simulink model "power_monophaseline"  (Simulink 6.0)
settings: Solver=ode23tb  SolverMode=SingleTasking  StartTime=0.0  StopTime=0.1  RelTol=1e-5  AbsTol=1e-5
libraries: powerlib x17
settings Model: Creator=patrice  LastModifiedBy=batserve  ExtModeTrigMode=oneshot  ExtModeArmWhenConnect=off  ExtModeAutoUpdateStatusClock=off
settings DataIOCC: LimitDataPoints=off  SaveOutput=off  SaveTime=off  SignalLoggingName=sigsOut
settings OptimizationCC: BlockReduction=off  BooleanDataType=off
settings DebuggingCC: CheckExecutionContextPreStartOutputMsg=on  CheckExecutionContextRuntimeOutputMsg=on  SolverPrmCheckMsg=none  IntegerOverflowMsg=none
settings HardwareCC: TargetUnknown=on
settings RTWCC: TemplateMakefile=grt_unix.tmf

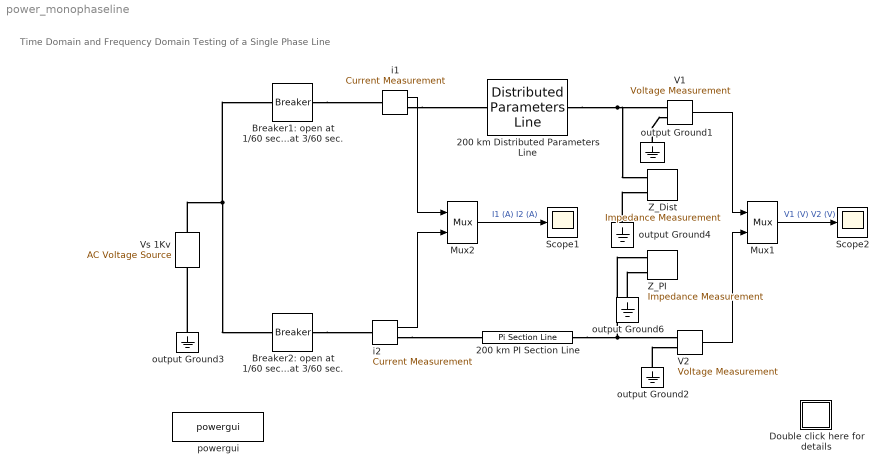
== system power_monophaseline ==
  note: Time Domain and Frequency Domain Testing of a Single Phase Line
  200 km Distributed Parameters Line : powerlib/Elements/Distributed Parameters Line  Phases=1  Frequency=60  Resistance=0.0955  Inductance=2.137e-3  Capacitance=12.37e-9  Length=200  x1=[0 -378.111478683995;0.000205658707571549 -305.271981817252;0.000411317415143098 -230.598373057679;0.000616976122714648 -154.539300699466;0.000822634830286197 -77.5517370737755;0.00102829353785775 -0.0982330023556983]  x2=[0 -417.766377531924;0.000205658707571549 -339.363445347372;0.000411317415143098 -258.921575532847;0.000616976122714648 -176.9240728097;0.000822634830286197 -93.8635883345532;0.00102829353785775 -10.2391597901105]  x3=[0 -1.7651045305041;0.000205658707571549 -1.62172775369337;0.000411317415143098 -1.4686074355911;0.000616976122714648 -1.30666354204152;0.000822634830286197 -1.13686905202344;0.00102829353785775 -0.960244111872024]  x4=[0 -0.971127277857831;0.000205658707571549 -0.788874156966986;0.000411317415143098 -0.601881382392148;0.000616976122714648 -0.411272429893128;0.000822634830286197 -0.218192501674784;0.00102829353785775 -0.0238016458702721]  x5=0.00102829353785775  Measurements=None
      settings: AttributesFormatString=\n
  200 km PI Section Line : powerlib/Elements/Pi Section Line  PhysicalDomain=powersysdomain  SubClassName=unknown  LeftPortType=p1  RightPortType=p1  LConnTagsString=__new0  RConnTagsString=__new0  Frequency=60  Resistance=0.0955  Inductance=2.137e-03  Capacitance=12.37e-09  Length=200  PiSections=2  Measurements=None
      settings: AttributesFormatString=\n
  Breaker1: open at 1/60 sec.  close at 3/60 sec. : powerlib/Elements/Breaker  BreakerResistance=0.1  InitialState=1  SnubberResistance=inf  SnubberCapacitance=0  SwitchingTimes="[ 1/60  3/60 ]"  External=off  Measurements=None
      settings: AttributesFormatString=\n
  Breaker2: open at 1/60 sec. close at 3/60 sec. : powerlib/Elements/Breaker  BreakerResistance=0.1  InitialState=1  SnubberResistance=inf  SnubberCapacitance=0  SwitchingTimes="[ 1/60  3/60 ]"  External=off  Measurements=None
      settings: AttributesFormatString=\n
  Double click here for details : Subsystem
      mask Display: disp('?')
  Mux1 : Mux  Inputs=2
  Mux2 : Mux  Inputs=2
  Scope1 : Scope
      settings: TickLabels=on  TimeRange=0.1  YMin=-4  YMax=4  DataFormat=Array
  Scope2 : Scope
      settings: TickLabels=on  TimeRange=0.1  YMin=-2500  YMax=2500  DataFormat=Array
  V1 : powerlib/Measurements/Voltage Measurement  Tag=PoWeRsYsTeMmEaSuReMeNt  PhasorSimulation=off  OutputType=Magnitude  PSBequivalent=0
  V2 : powerlib/Measurements/Voltage Measurement  Tag=PoWeRsYsTeMmEaSuReMeNt  PhasorSimulation=off  OutputType=Magnitude  PSBequivalent=0
  Vs 1Kv : powerlib/Electrical Sources/AC Voltage Source  Description=source block  Orientation=up  Amplitude=1e3  Phase=0  Frequency=60  SampleTime=0  Measurements=None
      settings: AttributesFormatString=\n
  Z_Dist : powerlib/Measurements/Impedance Measurement  PhysicalDomain=powersysdomain  SubClassName=unknown  LeftPortType=p1  RightPortType=p1  LConnTagsString=+|-  Factor=1
      settings: AttributesFormatString=\n
  Z_PI : powerlib/Measurements/Impedance Measurement  PhysicalDomain=powersysdomain  SubClassName=unknown  LeftPortType=p1  RightPortType=p1  LConnTagsString=+|-  Factor=1
      settings: AttributesFormatString=\n
  i1 : powerlib/Measurements/Current Measurement  Tag=PoWeRsYsTeMmEaSuReMeNt  PhasorSimulation=off  OutputType=Magnitude  PSBequivalent=0
  i2 : powerlib/Measurements/Current Measurement  Tag=PoWeRsYsTeMmEaSuReMeNt  PhasorSimulation=off  OutputType=Magnitude  PSBequivalent=0
  output Ground{1..4,6} (5 alike) : powerlib/Elements/Ground  Orientation=down  PhysicalDomain=powersysdomain  SubClassName=unknown  LeftPortType=p1  RightPortType=p1  LConnTagsString=a
  powergui : powerlib/powergui  Priority=2  Frange=0:2:2000  Ylog=on  Xlog=off  save=off  variable=ZData  ZoomFFT=on  StartTime=0.0  cycles=1  DisplayStyle=off  fundamental=60  FreqAxis=off  MaxFrequency=1000  frequencyindice=1  frequencyindicesteady=1  RmsSteady=1  display=on  Ts=0  methode=off  frequency=60  echomessages=on
  wires:
  Mux1/1 -> Scope2/1  "V1 (V) V2 (V)"
  Mux2/1 -> Scope1/1  "I1 (A) I2 (A)"
  i1/1 -> Mux2/1
  i2/1 -> Mux2/2
  V1/1 -> Mux1/1
  V2/1 -> Mux1/2
  connections:
  Breaker1: open at 1/60 sec.  close at 3/60 sec./RConn1 -- i1/LConn1
  i1/RConn1 -- 200 km Distributed Parameters Line/LConn1
  output Ground1/LConn1 -- V1/LConn2
  output Ground2/LConn1 -- V2/LConn2
  Breaker2: open at 1/60 sec. close at 3/60 sec./RConn1 -- i2/LConn1
  i2/RConn1 -- 200 km PI Section Line/LConn1
  output Ground3/LConn1 -- Vs 1Kv/LConn1
  Vs 1Kv/RConn1 -- Breaker1: open at 1/60 sec.  close at 3/60 sec./LConn1 -- Breaker2: open at 1/60 sec. close at 3/60 sec./LConn1
  200 km Distributed Parameters Line/RConn1 -- V1/LConn1 -- Z_Dist/LConn1
  output Ground4/LConn1 -- Z_Dist/LConn2
  output Ground6/LConn1 -- Z_PI/LConn2
  200 km PI Section Line/RConn1 -- V2/LConn1 -- Z_PI/LConn1

== system power_monophaseline/Double click here for details ==
  note: A  200 km line is connected on a 1 kV, 60 Hz  infinite source. The line is deenergized and then reenergized after 2 cycles.
      | The simulation is performed simultaneously with two different line models:
      |
      | - Distributed parameter line
      | - PI  section line consisting of two 100 km sections.
      |
      | Currents at the sending end and voltages at the receiving end are compared for the two line models.
      | Impedance Measurement blocks are connected at the open end of both  lines in order  to compare their frequency responses.
  note: Open the two scopes and start the simulation.
      | Observe the difference in current and voltage waveforms at breaker opening and reclosing.
      | Note the sharp edges of the distributed parameter model (in yellow).
      | These voltage and current steps which are due to travelling wave reflections at line ends are filtered by the PI model.
  note: Demonstration
  note: Circuit Description
  note: Open the Powergui block and select 'Steady-State Voltages and Currents' to display the voltage and current phasors.
      | Observe that the values obtained with the two models are the same.
  note: 2. Time domain comparison
  note: This demonstration compares time domain and frequencydomain performance
      | of distributed parameter line model and PI section line model
  note: 3. Frequency domain comparison
  note: Open  the Powergui block and select  'Impedance vs Frequency Measurement'.
      | A new window appears, listing the two Impedance Measurement blocks Z_Dist and Z_PI  connected to your circuit.
      | Note also that parameters are set to compute impedance in the 0:2000 Hz frequency range by steps of 2 Hz.
      | Using the 'CTRL' key, select both Z_Dist and Z_PI in the upper right window.
      | Then, click on the Display button.  The two impedances are computed and displayed on the same graph.
      |
      | Note that the distributed parameter line shows a succession of poles and zeros equally spaced, every 486 Hz.
      | The first pole occurs a 243 Hz , corresponding to frequency f = 1 / (4*T), where :
      |
      |          T = travelling time = length*sqrt(L*C) = 200*sqrt(2.137e-3*12.37e-9) = 1.028 ms
      |
      | The PI section line only shows two poles because it consists of two PI sections.
      | Impedance comparison shows that a two-PI line gives a good approximation
      | of the distributed line for the 0-350 Hz frequency range.
  note: 1. Steady-state
  note: G. Sybille (Hydro-Quebec)
